simulink model "Problem2"  (R2020b)
settings: Solver=VariableStepAuto  StartTime=0.0  StopTime=120  RelTol=1e-3
settings Model: Creator=Shirish  LastModifiedBy=Shirish

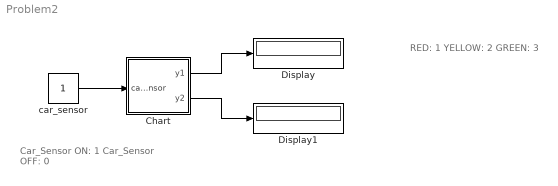
== system Problem2 ==
  note: RED: 1
      | YELLOW: 2
      | GREEN: 3
  note: Car_Sensor ON: 1
      | Car_Sensor OFF: 0
  Chart : Stateflow chart  TreatAsAtomicUnit=on
  Display : Display
  Display1 : Display
  car_sensor : Constant
  wires:
  Chart/1(y1) -> Display/1
  car_sensor/1 -> Chart/1(car_sensor)
  Chart/2(y2) -> Display1/1

== stateflow chart Problem2/Chart ==
  state Stop
    y1=red;
    y2=green;
  state StopForTraffic
    y1=red;
    y2=green;
  state StopToGo
    y1=red;
    y2=yellow;
  state GoToStop
    y1=yellow;
    y2=red;
  state Go
    y1=green;
    y2=red;
  (default) -> Stop
  Stop -> StopForTraffic : after(20,tick)
  StopForTraffic -> StopToGo : [car_sensor]
  GoToStop -> Stop : after(3,tick)
  StopToGo -> Go : after(3,tick)
  Go -> GoToStop : after(10,tick)
  data: green constant double =3; yellow constant double =2; red constant double =1; y1 output; car_sensor input; y2 output
